simulink model "vsi_fmt_core"  (Simulink 7.0)
settings: Solver=ode45  StartTime=0.0  StopTime=10.0  RelTol=1e-3
libraries: xbsIndex_r4 x293, xbsReplacements_r4 x15, simulink x3, vlbi_lib x1
(part 1 of 2)
settings Model: Creator=mdexter  LastModifiedBy=mdexter

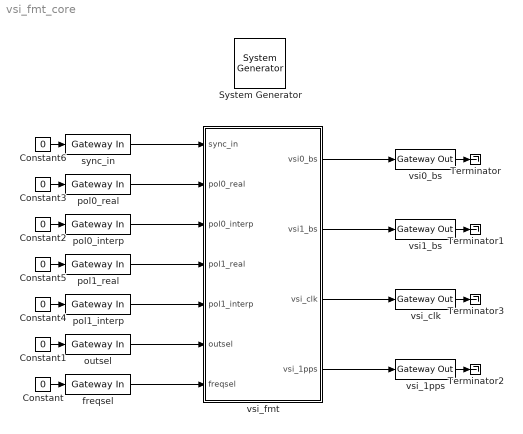
== system vsi_fmt_core ==
  " System Generator" : xbsIndex_r4/ System Generator  Tag=genX  SystemSampleTime=-1  xilinxfamily=virtex2p  part=xc2vp50  speed=-7  package=ff1152  synthesis_tool=XST  clock_wrapper=Clock Enables  directory=./vsi_fmt_core  testbench=off  simulink_period=1  sysclk_period=100  dcm_input_clock_period=100  incr_netlist=off  trim_vbits=Everywhere in SubSystem  dbl_ovrd=According to Block Masks  core_generation=According to Block Masks  run_coregen=off  deprecated_control=off  eval_field=0  block_type=sysgen
      settings: block_version=10.1.3
  Constant{,1..6} (7 alike) : Constant  Value=0
  Terminator{,1..3} (4 alike) : Terminator
  freqsel : xbsIndex_r4/Gateway In  arith_type=Unsigned  n_bits=3  bin_pt=0  quantization="Round  (unbiased: +/- Inf)"  overflow=Saturate  period=1  dbl_ovrd=off  timing_constraint=None  locs_specified=off  LOCs={}  block_type=gatewayin
      settings: infoedit="Gateway in block.  Converts inputs of type Simulink integer, double and fixed point to  Xilinx fixed point type.<P><P>Hardware notes:  In hardware these blocks become top level input ports."  block_version=10.1.3
  outsel : xbsIndex_r4/Gateway In  arith_type=Unsigned  n_bits=2  bin_pt=0  quantization="Round  (unbiased: +/- Inf)"  overflow=Saturate  period=1  dbl_ovrd=off  timing_constraint=None  locs_specified=off  LOCs={}  block_type=gatewayin
      settings: infoedit="Gateway in block.  Converts inputs of type Simulink integer, double and fixed point to  Xilinx fixed point type.<P><P>Hardware notes:  In hardware these blocks become top level input ports."  block_version=10.1.3
  pol0_interp : xbsIndex_r4/Gateway In  arith_type=Unsigned  n_bits=4  bin_pt=0  quantization="Round  (unbiased: +/- Inf)"  overflow=Saturate  period=1  dbl_ovrd=off  timing_constraint=None  locs_specified=off  LOCs={}  block_type=gatewayin
      settings: infoedit="Gateway in block.  Converts inputs of type Simulink integer, double and fixed point to  Xilinx fixed point type.<P><P>Hardware notes:  In hardware these blocks become top level input ports."  block_version=10.1.3
  pol0_real : xbsIndex_r4/Gateway In  arith_type=Unsigned  n_bits=4  bin_pt=0  quantization="Round  (unbiased: +/- Inf)"  overflow=Saturate  period=1  dbl_ovrd=off  timing_constraint=None  locs_specified=off  LOCs={}  block_type=gatewayin
      settings: infoedit="Gateway in block.  Converts inputs of type Simulink integer, double and fixed point to  Xilinx fixed point type.<P><P>Hardware notes:  In hardware these blocks become top level input ports."  block_version=10.1.3
  pol1_interp : xbsIndex_r4/Gateway In  arith_type=Unsigned  n_bits=4  bin_pt=0  quantization="Round  (unbiased: +/- Inf)"  overflow=Saturate  period=1  dbl_ovrd=off  timing_constraint=None  locs_specified=off  LOCs={}  block_type=gatewayin
      settings: infoedit="Gateway in block.  Converts inputs of type Simulink integer, double and fixed point to  Xilinx fixed point type.<P><P>Hardware notes:  In hardware these blocks become top level input ports."  block_version=10.1.3
  pol1_real : xbsIndex_r4/Gateway In  arith_type=Unsigned  n_bits=4  bin_pt=0  quantization="Round  (unbiased: +/- Inf)"  overflow=Saturate  period=1  dbl_ovrd=off  timing_constraint=None  locs_specified=off  LOCs={}  block_type=gatewayin
      settings: infoedit="Gateway in block.  Converts inputs of type Simulink integer, double and fixed point to  Xilinx fixed point type.<P><P>Hardware notes:  In hardware these blocks become top level input ports."  block_version=10.1.3
  sync_in : xbsIndex_r4/Gateway In  arith_type=Boolean  n_bits=16  bin_pt=14  quantization="Round  (unbiased: +/- Inf)"  overflow=Saturate  period=1  dbl_ovrd=off  timing_constraint=None  locs_specified=off  LOCs={}  block_type=gatewayin
      settings: infoedit="Gateway in block.  Converts inputs of type Simulink integer, double and fixed point to  Xilinx fixed point type.<P><P>Hardware notes:  In hardware these blocks become top level input ports."  block_version=10.1.3
  vsi0_bs : xbsIndex_r4/Gateway Out  hdl_port=on  timing_constraint=None  locs_specified=off  LOCs={}  block_type=gatewayout
      settings: infoedit="Gateway out block.  Converts Xilinx fixed point inputs into ouputs of type Simulink integer, double, or fixed point.<P><P>Hardware notes:  In hardware these blocks become top level output ports or are discarded, depending on how they are configured."  block_version=10.1.3
  vsi1_bs : xbsIndex_r4/Gateway Out  hdl_port=on  timing_constraint=None  locs_specified=off  LOCs={}  block_type=gatewayout
      settings: infoedit="Gateway out block.  Converts Xilinx fixed point inputs into ouputs of type Simulink integer, double, or fixed point.<P><P>Hardware notes:  In hardware these blocks become top level output ports or are discarded, depending on how they are configured."  block_version=10.1.3
  vsi_1pps : xbsIndex_r4/Gateway Out  hdl_port=on  timing_constraint=None  locs_specified=off  LOCs={}  block_type=gatewayout
      settings: infoedit="Gateway out block.  Converts Xilinx fixed point inputs into ouputs of type Simulink integer, double, or fixed point.<P><P>Hardware notes:  In hardware these blocks become top level output ports or are discarded, depending on how they are configured."  block_version=10.1.3
  vsi_clk : xbsIndex_r4/Gateway Out  hdl_port=on  timing_constraint=None  locs_specified=off  LOCs={}  block_type=gatewayout
      settings: infoedit="Gateway out block.  Converts Xilinx fixed point inputs into ouputs of type Simulink integer, double, or fixed point.<P><P>Hardware notes:  In hardware these blocks become top level output ports or are discarded, depending on how they are configured."  block_version=10.1.3
  vsi_fmt : Subsystem
  wires:
  vsi_fmt/1(vsi0_bs) -> vsi0_bs/1
  pol0_real/1 -> vsi_fmt/2(pol0_real)
  vsi_fmt/2(vsi1_bs) -> vsi1_bs/1
  pol1_real/1 -> vsi_fmt/4(pol1_real)
  pol0_interp/1 -> vsi_fmt/3(pol0_interp)
  pol1_interp/1 -> vsi_fmt/5(pol1_interp)
  sync_in/1 -> vsi_fmt/1(sync_in)
  outsel/1 -> vsi_fmt/6(outsel)
  vsi_fmt/3(vsi_clk) -> vsi_clk/1
  vsi_fmt/4(vsi_1pps) -> vsi_1pps/1
  freqsel/1 -> vsi_fmt/7(freqsel)
  Constant/1 -> freqsel/1
  Constant1/1 -> outsel/1
  Constant2/1 -> pol0_interp/1
  Constant3/1 -> pol0_real/1
  Constant4/1 -> pol1_interp/1
  Constant5/1 -> pol1_real/1
  Constant6/1 -> sync_in/1
  vsi0_bs/1 -> Terminator/1
  vsi1_bs/1 -> Terminator1/1
  vsi_1pps/1 -> Terminator2/1
  vsi_clk/1 -> Terminator3/1

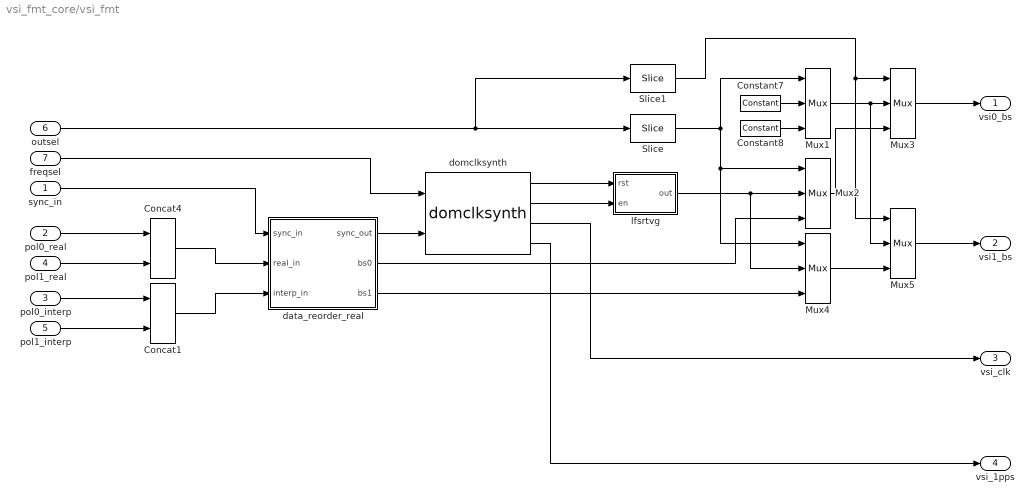
== system vsi_fmt_core/vsi_fmt ==
  sync_in : Inport  OutDataType=sfix(16)  OutScaling=2^0
  pol0_real : Inport  Port=2  OutDataType=sfix(16)  OutScaling=2^0
  pol0_interp : Inport  Port=3  OutDataType=sfix(16)  OutScaling=2^0
  pol1_real : Inport  Port=4  OutDataType=sfix(16)  OutScaling=2^0
  pol1_interp : Inport  Port=5  OutDataType=sfix(16)  OutScaling=2^0
  outsel : Inport  Port=6  OutDataType=sfix(16)  OutScaling=2^0
  freqsel : Inport  Port=7  OutDataType=sfix(16)  OutScaling=2^0
  Concat1 : xbsIndex_r4/Concat  num_inputs=2  dbl_ovrd=off  block_type=concat
      settings: block_version=11.3
  Concat4 : xbsIndex_r4/Concat  num_inputs=2  dbl_ovrd=off  block_type=concat
      settings: block_version=11.3
  Constant7 : xbsIndex_r4/Constant  arith_type=Unsigned  const=0  n_bits=32  bin_pt=0  explicit_period=on  period=1  equ=P=C  opselect=C  inp2=PCIN>>17  opr=+  inp1=P  carry=CIN  dbl_ovrd=off  block_type=constant
      settings: block_version=11.3
  Constant8 : xbsIndex_r4/Constant  arith_type=Unsigned  const=2^32-1  n_bits=32  bin_pt=0  explicit_period=on  period=1  equ=P=C  opselect=C  inp2=PCIN>>17  opr=+  inp1=P  carry=CIN  dbl_ovrd=off  block_type=constant
      settings: block_version=11.3
  Mux{1..5} (5 alike) : xbsIndex_r4/Mux  inputs=2  en=off  latency=1  precision=Full  arith_type="Signed  (2's comp)"  n_bits=8  bin_pt=2  quantization=Truncate  overflow=Wrap  dbl_ovrd=off  block_type=mux
      settings: xl_area=[0, 0, 0, 0, 0, 0, 0]  block_version=11.3
  Slice : xbsIndex_r4/Slice  nbits=1  boolean_output=off  mode=Lower Bit Location + Width  bit1=0  base1=MSB of Input  bit0=0  base0=LSB of Input  dbl_ovrd=off  block_type=slice
      settings: block_version=11.3
  Slice1 : xbsIndex_r4/Slice  nbits=1  boolean_output=off  mode=Lower Bit Location + Width  bit1=0  base1=MSB of Input  bit0=1  base0=LSB of Input  dbl_ovrd=off  block_type=slice
      settings: block_version=11.3
  data_reorder_real : Subsystem  mask{sample_width=2, vsi_clock=64 MHz}
      mask prompts: sample_width "Channel sample width:"; vsi_clock "VSI output clock rate:"
      mask init:
      | myname = gcb;
      | 
      | if (strcmp(vsi_clock, '32 MHz'))
      |     set_param([gcb, '/restream'], 'clock_rate', '32');
      |     set_param([gcb, '/slc_wrmask'], 'bit1', '-1');
      | else
      |     set_param([gcb, '/restream'], 'clock_rate', '64');
      |     set_param([gcb, '/slc_wrmask'], 'bit1', '0');
      | end
      mask StyleString: edit,popup(32 MHz|64 MHz)
  domclksynth : vlbi_lib/domclksynth  SystemSampleTime=-1
  lfsrtvg : Subsystem
  vsi0_bs : Outport  OutDataType=sfix(16)  OutScaling=2^0
  vsi1_bs : Outport  Port=2  OutDataType=sfix(16)  OutScaling=2^0
  vsi_clk : Outport  Port=3  OutDataType=sfix(16)  OutScaling=2^0
  vsi_1pps : Outport  Port=4  OutDataType=sfix(16)  OutScaling=2^0
  wires:
  domclksynth/2 -> lfsrtvg/2(en)
  domclksynth/3 -> vsi_clk/1
  domclksynth/4 -> vsi_1pps/1
  data_reorder_real/1(sync_out) -> domclksynth/2
  data_reorder_real/2(bs0) -> Mux2/3
  domclksynth/1 -> lfsrtvg/1(rst)
  outsel/1 -> Slice/1, Slice1/1
  Constant7/1 -> Mux1/2
  Constant8/1 -> Mux1/3
  Slice/1 -> Mux1/1, Mux2/1, Mux4/1
  lfsrtvg/1(out) -> Mux2/2, Mux4/2
  Mux1/1 -> Mux3/2, Mux5/2
  Mux2/1 -> Mux3/3
  Slice1/1 -> Mux3/1, Mux5/1
  Concat4/1 -> data_reorder_real/2(real_in)
  Concat1/1 -> data_reorder_real/3(interp_in)
  data_reorder_real/3(bs1) -> Mux4/3
  Mux4/1 -> Mux5/3
  pol0_real/1 -> Concat4/1
  pol1_real/1 -> Concat4/2
  pol0_interp/1 -> Concat1/1
  pol1_interp/1 -> Concat1/2
  sync_in/1 -> data_reorder_real/1(sync_in)
  Mux3/1 -> vsi0_bs/1
  Mux5/1 -> vsi1_bs/1
  freqsel/1 -> domclksynth/1

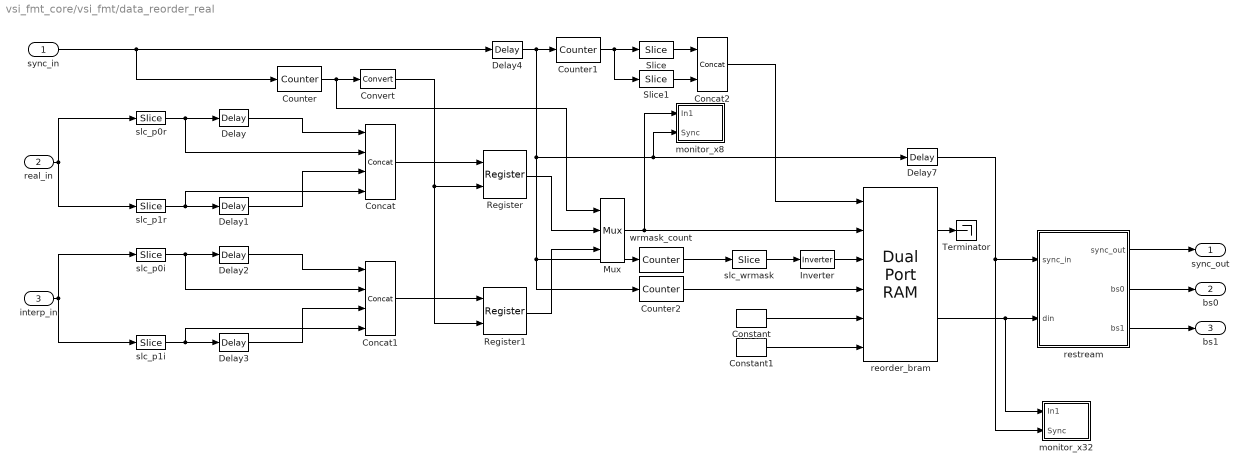
== system vsi_fmt_core/vsi_fmt/data_reorder_real ==
  sync_in : Inport  OutDataType=sfix(16)  OutScaling=2^0
  real_in : Inport  Port=2  OutDataType=sfix(16)  OutScaling=2^0
  interp_in : Inport  Port=3  OutDataType=sfix(16)  OutScaling=2^0
  Concat : xbsIndex_r4/Concat  num_inputs=4  dbl_ovrd=off  block_type=concat
      settings: block_version=11.3
  Concat1 : xbsIndex_r4/Concat  num_inputs=4  dbl_ovrd=off  block_type=concat
      settings: block_version=11.3
  Concat2 : xbsIndex_r4/Concat  num_inputs=2  dbl_ovrd=off  block_type=concat
      settings: block_version=11.3
  Constant : xbsIndex_r4/Constant  arith_type=Unsigned  const=0  n_bits=32*sample_width  bin_pt=0  explicit_period=on  period=1  equ=P=C  opselect=C  inp2=PCIN>>17  opr=+  inp1=P  carry=CIN  dbl_ovrd=off  block_type=constant
      settings: block_version=11.3
  Constant1 : xbsIndex_r4/Constant  arith_type=Boolean  const=0  n_bits=8*sample_width  bin_pt=0  explicit_period=on  period=1  equ=P=C  opselect=C  inp2=PCIN>>17  opr=+  inp1=P  carry=CIN  dbl_ovrd=off  block_type=constant
      settings: block_version=11.3
  Convert : xbsIndex_r4/Convert  arith_type=Boolean  n_bits=8  bin_pt=6  quantization=Truncate  overflow=Wrap  latency=0  dbl_ovrd=off  pipeline=off  block_type=convert
      settings: xl_area=[0, 0, 0, 0, 0, 0, 0]  block_version=11.3
  Counter : xbsIndex_r4/Counter  cnt_type=Free Running  cnt_to=Inf  operation=Up  start_count=0  cnt_by_val=1  arith_type=Unsigned  n_bits=1  bin_pt=0  load_pin=off  rst=on  en=off  explicit_period=off  period=1  dbl_ovrd=off  use_behavioral_HDL=off  use_rpm=on  implementation=Fabric  block_type=counter
      settings: xl_area=[0, 0, 0, 0, 0, 0, 0]  block_version=11.3
  Counter1 : xbsIndex_r4/Counter  cnt_type=Free Running  cnt_to=Inf  operation=Up  start_count=0  cnt_by_val=1  arith_type=Unsigned  n_bits=3  bin_pt=0  load_pin=off  rst=on  en=off  explicit_period=off  period=1  dbl_ovrd=off  use_behavioral_HDL=off  use_rpm=on  implementation=Fabric  block_type=counter
      settings: xl_area=[0, 0, 0, 0, 0, 0, 0]  block_version=11.3
  Counter2 : xbsIndex_r4/Counter  cnt_type=Free Running  cnt_to=Inf  operation=Up  start_count=0  cnt_by_val=1  arith_type=Unsigned  n_bits=1  bin_pt=0  load_pin=off  rst=on  en=off  explicit_period=off  period=1  dbl_ovrd=off  use_behavioral_HDL=off  use_rpm=on  implementation=Fabric  block_type=counter
      settings: xl_area=[0, 0, 0, 0, 0, 0, 0]  block_version=11.3
  Delay{,1..3} (4 alike) : xbsIndex_r4/Delay  en=off  latency=1  dbl_ovrd=off  reg_retiming=off  block_type=delay
      settings: xl_area=[0, 0, 0, 0, 0, 0, 0]  block_version=11.3
  Delay4 : xbsIndex_r4/Delay  en=off  latency=3  dbl_ovrd=off  reg_retiming=off  block_type=delay
      settings: xl_area=[0, 0, 0, 0, 0, 0, 0]  block_version=11.3
  Delay7 : xbsIndex_r4/Delay  en=off  latency=11  dbl_ovrd=off  reg_retiming=off  block_type=delay
      settings: xl_area=[0, 0, 0, 0, 0, 0, 0]  block_version=11.3
  Inverter : xbsIndex_r4/Inverter  en=off  latency=0  dbl_ovrd=off  block_type=inv
      settings: xl_area=[0, 0, 0, 0, 0, 0, 0]  block_version=11.3
  Mux : xbsIndex_r4/Mux  inputs=2  en=off  latency=1  precision=Full  arith_type="Signed  (2's comp)"  n_bits=8  bin_pt=2  quantization=Truncate  overflow=Wrap  dbl_ovrd=off  block_type=mux
      settings: xl_area=[0, 0, 0, 0, 0, 0, 0]  block_version=11.3
  Register : xbsIndex_r4/Register  init=0  rst=off  en=on  dbl_ovrd=off  block_type=register
      settings: xl_area=[0, 0, 0, 0, 0, 0, 0]  block_version=11.3
  Register1 : xbsIndex_r4/Register  init=0  rst=off  en=on  dbl_ovrd=off  block_type=register
      settings: xl_area=[0, 0, 0, 0, 0, 0, 0]  block_version=11.3
  Slice : xbsIndex_r4/Slice  nbits=1  boolean_output=off  mode=Lower Bit Location + Width  bit1=0  base1=MSB of Input  bit0=0  base0=LSB of Input  dbl_ovrd=off  block_type=slice
      settings: block_version=11.3
  Slice1 : xbsIndex_r4/Slice  nbits=2  boolean_output=off  mode=Upper Bit Location + Width  bit1=0  base1=MSB of Input  bit0=0  base0=LSB of Input  dbl_ovrd=off  block_type=slice
      settings: block_version=11.3
  Terminator : Terminator
  monitor_x32 : Subsystem
  monitor_x8 : Subsystem
  reorder_bram : xbsIndex_r4/Dual Port RAM  depth=8  initVector=zeros(2)  distributed_mem=Block RAM  init_a=0  init_b=0  rst_a=off  rst_b=off  en_a=off  en_b=off  latency=3  write_mode_A=Read Before Write  write_mode_B=Read Before Write  dbl_ovrd=off  optimize=Area  use_rpm=off  block_type=dpram
      settings: xl_area=[0, 0, 0, 0, 0, 0, 0]  block_version=11.3
  restream : Subsystem  mask{clock_rate=64}
      mask prompts: clock_rate "Clock rate (MHz)"
  slc_p0i : xbsIndex_r4/Slice  nbits=2*sample_width  boolean_output=off  mode=Upper Bit Location + Width  bit1=0  base1=MSB of Input  bit0=0  base0=LSB of Input  dbl_ovrd=off  block_type=slice
      settings: block_version=11.3
  slc_p0r : xbsIndex_r4/Slice  nbits=2*sample_width  boolean_output=off  mode=Upper Bit Location + Width  bit1=0  base1=MSB of Input  bit0=0  base0=LSB of Input  dbl_ovrd=off  block_type=slice
      settings: block_version=11.3
  slc_p1i : xbsIndex_r4/Slice  nbits=2*sample_width  boolean_output=off  mode=Upper Bit Location + Width  bit1=-2*sample_width  base1=MSB of Input  bit0=0  base0=LSB of Input  dbl_ovrd=off  block_type=slice
      settings: block_version=11.3
  slc_p1r : xbsIndex_r4/Slice  nbits=2*sample_width  boolean_output=off  mode=Upper Bit Location + Width  bit1=-2*sample_width  base1=MSB of Input  bit0=0  base0=LSB of Input  dbl_ovrd=off  block_type=slice
      settings: block_version=11.3
  slc_wrmask : xbsIndex_r4/Slice  nbits=1  boolean_output=on  mode=Upper Bit Location + Width  bit1=0  base1=MSB of Input  bit0=0  base0=LSB of Input  dbl_ovrd=off  block_type=slice
      settings: block_version=11.3
  wrmask_count : xbsIndex_r4/Counter  cnt_type=Count Limited  cnt_to=31  operation=Up  start_count=0  cnt_by_val=1  arith_type=Unsigned  n_bits=6  bin_pt=0  load_pin=off  rst=on  en=off  explicit_period=off  period=1  dbl_ovrd=off  use_behavioral_HDL=off  use_rpm=on  implementation=Fabric  block_type=counter
      settings: xl_area=[0, 0, 0, 0, 0, 0, 0]  block_version=11.3
  sync_out : Outport  OutDataType=sfix(16)  OutScaling=2^0
  bs0 : Outport  Port=2  OutDataType=sfix(16)  OutScaling=2^0
  bs1 : Outport  Port=3  OutDataType=sfix(16)  OutScaling=2^0
  wires:
  Inverter/1 -> reorder_bram/3
  wrmask_count/1 -> slc_wrmask/1
  restream/3(bs1) -> bs1/1
  restream/2(bs0) -> bs0/1
  restream/1(sync_out) -> sync_out/1
  reorder_bram/2 -> monitor_x32/1(In1), restream/2(din)
  Delay7/1 -> monitor_x32/2(Sync), restream/1(sync_in)
  Concat2/1 -> reorder_bram/1
  Counter1/1 -> Slice1/1, Slice/1
  Slice1/1 -> Concat2/2
  Slice/1 -> Concat2/1
  reorder_bram/1 -> Terminator/1
  Counter2/1 -> reorder_bram/4
  Delay4/1 -> wrmask_count/1, Counter2/1, monitor_x8/2(Sync), Delay7/1, Counter1/1
  slc_wrmask/1 -> Inverter/1
  Mux/1 -> reorder_bram/2, monitor_x8/1(In1)
  Constant1/1 -> reorder_bram/6
  Constant/1 -> reorder_bram/5
  Register1/1 -> Mux/3
  Register/1 -> Mux/2
  Convert/1 -> Register1/2, Register/2
  Counter/1 -> Mux/1, Convert/1
  sync_in/1 -> Delay4/1, Counter/1
  Concat1/1 -> Register1/1
  Concat/1 -> Register/1
  Delay3/1 -> Concat1/3
  Delay2/1 -> Concat1/1
  Delay1/1 -> Concat/3
  Delay/1 -> Concat/1
  slc_p1i/1 -> Concat1/4, Delay3/1
  slc_p0i/1 -> Concat1/2, Delay2/1
  slc_p1r/1 -> Concat/4, Delay1/1
  slc_p0r/1 -> Concat/2, Delay/1
  interp_in/1 -> slc_p1i/1, slc_p0i/1
  real_in/1 -> slc_p1r/1, slc_p0r/1

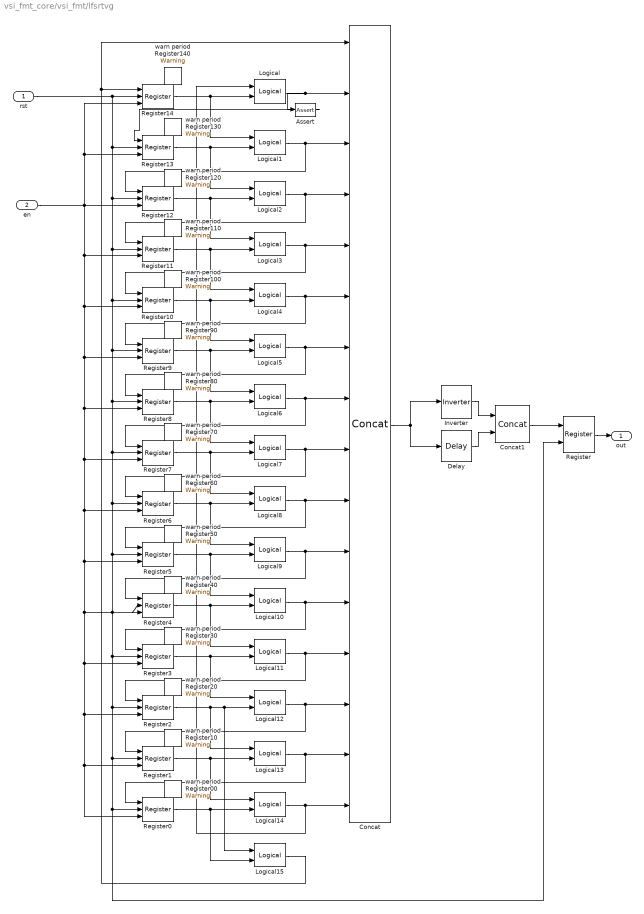
== system vsi_fmt_core/vsi_fmt/lfsrtvg ==
  rst : Inport  OutDataType=sfix(16)  OutScaling=2^0
  en : Inport  Port=2  OutDataType=sfix(16)  OutScaling=2^0
  Assert : xbsIndex_r4/Assert  assert_type=on  type_source=Explicitly  arith_type=Boolean  n_bits=16  bin_pt=14  assert_rate=on  rate_source=Explicitly  period=1  output_port=on  block_type=assert
      settings: block_version=11.3
  Concat : xbsIndex_r4/Concat  num_inputs=16  dbl_ovrd=off  block_type=concat
      settings: block_version=11.3
  Concat1 : xbsIndex_r4/Concat  num_inputs=2  dbl_ovrd=off  block_type=concat
      settings: block_version=11.3
  Delay : xbsIndex_r4/Delay  en=off  latency=0  dbl_ovrd=off  reg_retiming=off  block_type=delay
      settings: xl_area=[0, 0, 0, 0, 0, 0, 0]  block_version=11.3
  Inverter : xbsIndex_r4/Inverter  en=off  latency=0  dbl_ovrd=off  block_type=inv
      settings: xl_area=[0, 0, 0, 0, 0, 0, 0]  block_version=11.3
  Logical{,1..15} (16 alike) : xbsIndex_r4/Logical  logical_function=XOR  inputs=2  en=off  latency=0  precision=Full  arith_type=Unsigned  n_bits=8  bin_pt=2  align_bp=on  dbl_ovrd=off  block_type=logical
      settings: xl_area=[0, 0, 0, 0, 0, 0, 0]  block_version=11.3
  Register : xbsIndex_r4/Register  init=3221176320  rst=on  en=off  dbl_ovrd=off  block_type=register
      settings: xl_area=[0, 0, 0, 0, 0, 0, 0]  block_version=11.3
  Register{0..14} (15 alike) : xbsIndex_r4/Register  init=1  rst=on  en=on  dbl_ovrd=off  block_type=register
      settings: xl_area=[0, 0, 0, 0, 0, 0, 0]  block_version=11.3
  warn period Register00 : xbsReplacements_r4/Warning  SystemSampleTime=-1  period=1
  warn period Register{10,20,30,40,50,60,70,80,90,100,110,120,130,140} (14 alike) : xbsReplacements_r4/Warning  SystemSampleTime=-1  period=1
  out : Outport  OutDataType=sfix(16)  OutScaling=2^0
  wires:
  en/1 -> Register9/3, Register8/3, Register0/3, Register1/3, Register2/3, Register3/3, Register4/3, Register5/3, Register6/3, Register7/3, Register10/3, Register11/3, Register12/3, Register13/3, Register14/3
  rst/1 -> Register13/2, Register12/2, Register11/2, Register10/2, Register9/2, Register8/2, Register7/2, Register6/2, Register5/2, Register4/2, Register3/2, Register2/2, Register1/2, Register0/2, Register/2, Register14/2
  Register14/1 -> Logical1/1, Logical/2
  Register13/1 -> Logical2/1, Logical1/2
  Register12/1 -> Logical3/1, Logical2/2
  Register11/1 -> Logical4/1, Logical3/2
  Register10/1 -> Logical5/1, Logical4/2
  Register9/1 -> Logical6/1, Logical5/2
  Register8/1 -> Logical7/1, Logical6/2
  Register7/1 -> Logical8/1, Logical7/2
  Register6/1 -> Logical9/1, Logical8/2
  Register5/1 -> Logical10/1, Logical9/2
  Register4/1 -> Logical11/1, Logical10/2
  Register3/1 -> Logical12/1, Logical11/2
  Register2/1 -> Logical13/1, Logical12/2, Logical15/1
  Register1/1 -> Logical14/1, Logical13/2
  Register0/1 -> Logical14/2, Logical15/2
  Logical14/1 -> Logical/1, Concat/16
  Logical15/1 -> Register14/1, Concat/1
  Logical/1 -> Concat/2, Assert/1
  Logical1/1 -> Register12/1, Concat/3
  Logical2/1 -> Register11/1, Concat/4
  Logical3/1 -> Register10/1, Concat/5
  Logical4/1 -> Register9/1, Concat/6
  Logical5/1 -> Register8/1, Concat/7
  Logical6/1 -> Register7/1, Concat/8
  Logical7/1 -> Register6/1, Concat/9
  Logical8/1 -> Register5/1, Concat/10
  Logical9/1 -> Register4/1, Concat/11
  Logical10/1 -> Register3/1, Concat/12
  Logical11/1 -> Register2/1, Concat/13
  Logical12/1 -> Register1/1, Concat/14
  Logical13/1 -> Register0/1, Concat/15
  Concat/1 -> Inverter/1, Delay/1
  Inverter/1 -> Concat1/1
  Delay/1 -> Concat1/2
  Concat1/1 -> Register/1
  Register/1 -> out/1
  Assert/1 -> Register13/1

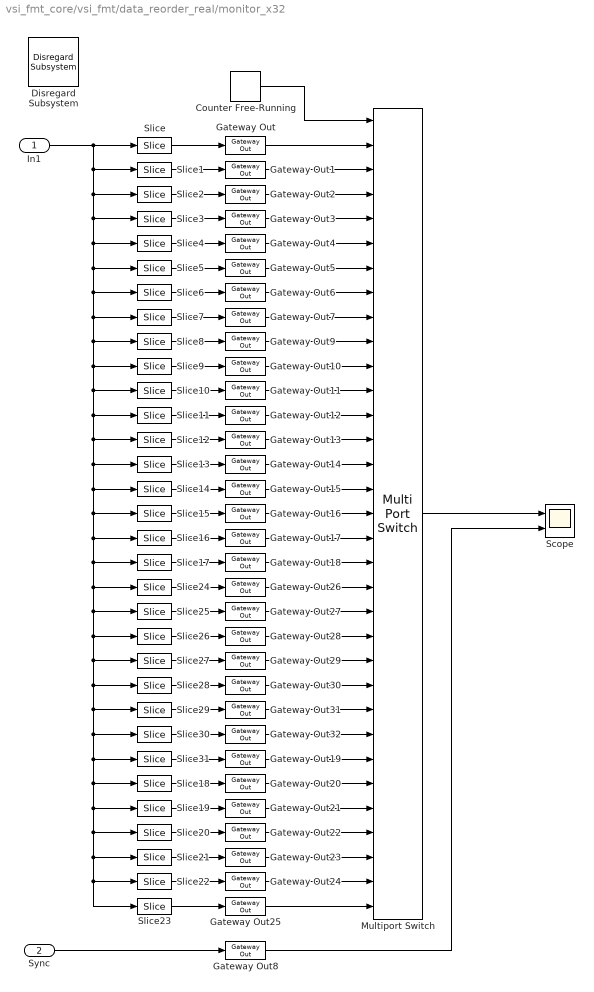
== system vsi_fmt_core/vsi_fmt/data_reorder_real/monitor_x32 ==
  In1 : Inport  OutDataType=sfix(16)  OutScaling=2^0
  Sync : Inport  Port=2  OutDataType=sfix(16)  OutScaling=2^0
  Counter Free-Running : simulink/Sources/Counter Free-Running  SystemSampleTime=-1  NumBits=5  tsamp=1/32
  Disregard Subsystem : xbsIndex_r4/Disregard Subsystem  Tag=discardX  block_type=disregard
      settings: block_version=11.3
  Gateway Out{,1..32} (33 alike) : xbsIndex_r4/Gateway Out  hdl_port=off  timing_constraint=None  locs_specified=off  LOCs={}  block_type=gatewayout
      settings: infoedit="Gateway out block.  Converts Xilinx fixed point inputs into ouputs of type Simulink integer, double, or fixed point.<br><br>Hardware notes:  In hardware these blocks become top level output ports or are discarded, depending on how they are configured."  xl_area=[0, 0, 0, 0, 0, 0, 0]  block_version=11.3
  Multiport Switch : MultiPortSwitch  Inputs=32  zeroidx=on  SampleTime=1/32
  Scope : Scope  NumInputPorts=2
      settings: YMin=-5~-5  YMax=5~5
  Slice : xbsIndex_r4/Slice  nbits=sample_width  boolean_output=off  mode=Lower Bit Location + Width  bit1=sample_width*0  base1=MSB of Input  bit0=sample_width*7  base0=LSB of Input  dbl_ovrd=off  block_type=slice
      settings: block_version=11.3
  Slice1 : xbsIndex_r4/Slice  nbits=sample_width  boolean_output=off  mode=Lower Bit Location + Width  bit1=-2*sample_width  base1=MSB of Input  bit0=sample_width*6  base0=LSB of Input  dbl_ovrd=off  block_type=slice
      settings: block_version=11.3
  Slice10 : xbsIndex_r4/Slice  nbits=sample_width  boolean_output=off  mode=Lower Bit Location + Width  bit1=sample_width*21  base1=MSB of Input  bit0=sample_width*21  base0=LSB of Input  dbl_ovrd=off  block_type=slice
      settings: block_version=11.3
  Slice11 : xbsIndex_r4/Slice  nbits=sample_width  boolean_output=off  mode=Lower Bit Location + Width  bit1=-22*sample_width  base1=MSB of Input  bit0=sample_width*20  base0=LSB of Input  dbl_ovrd=off  block_type=slice
      settings: block_version=11.3
  Slice12 : xbsIndex_r4/Slice  nbits=sample_width  boolean_output=off  mode=Lower Bit Location + Width  bit1=-24*sample_width  base1=MSB of Input  bit0=sample_width*31  base0=LSB of Input  dbl_ovrd=off  block_type=slice
      settings: block_version=11.3
  Slice13 : xbsIndex_r4/Slice  nbits=sample_width  boolean_output=off  mode=Lower Bit Location + Width  bit1=-26*sample_width  base1=MSB of Input  bit0=sample_width*30  base0=LSB of Input  dbl_ovrd=off  block_type=slice
      settings: block_version=11.3
  Slice14 : xbsIndex_r4/Slice  nbits=sample_width  boolean_output=off  mode=Lower Bit Location + Width  bit1=-28*sample_width  base1=MSB of Input  bit0=sample_width*29  base0=LSB of Input  dbl_ovrd=off  block_type=slice
      settings: block_version=11.3
  Slice15 : xbsIndex_r4/Slice  nbits=sample_width  boolean_output=off  mode=Lower Bit Location + Width  bit1=-30*sample_width  base1=MSB of Input  bit0=sample_width*28  base0=LSB of Input  dbl_ovrd=off  block_type=slice
      settings: block_version=11.3
  Slice16 : xbsIndex_r4/Slice  nbits=sample_width  boolean_output=off  mode=Lower Bit Location + Width  bit1=-1*sample_width  base1=MSB of Input  bit0=sample_width*3  base0=LSB of Input  dbl_ovrd=off  block_type=slice
      settings: block_version=11.3
  Slice17 : xbsIndex_r4/Slice  nbits=sample_width  boolean_output=off  mode=Lower Bit Location + Width  bit1=-3*sample_width  base1=MSB of Input  bit0=sample_width*2  base0=LSB of Input  dbl_ovrd=off  block_type=slice
      settings: block_version=11.3
  Slice18 : xbsIndex_r4/Slice  nbits=sample_width  boolean_output=off  mode=Lower Bit Location + Width  bit1=-21*sample_width  base1=MSB of Input  bit0=sample_width*17  base0=LSB of Input  dbl_ovrd=off  block_type=slice
      settings: block_version=11.3
  Slice19 : xbsIndex_r4/Slice  nbits=sample_width  boolean_output=off  mode=Lower Bit Location + Width  bit1=-23*sample_width  base1=MSB of Input  bit0=sample_width*16  base0=LSB of Input  dbl_ovrd=off  block_type=slice
      settings: block_version=11.3
  Slice2 : xbsIndex_r4/Slice  nbits=sample_width  boolean_output=off  mode=Lower Bit Location + Width  bit1=-4*sample_width  base1=MSB of Input  bit0=sample_width*5  base0=LSB of Input  dbl_ovrd=off  block_type=slice
      settings: block_version=11.3
  Slice20 : xbsIndex_r4/Slice  nbits=sample_width  boolean_output=off  mode=Lower Bit Location + Width  bit1=-25*sample_width  base1=MSB of Input  bit0=sample_width*27  base0=LSB of Input  dbl_ovrd=off  block_type=slice
      settings: block_version=11.3
  Slice21 : xbsIndex_r4/Slice  nbits=sample_width  boolean_output=off  mode=Lower Bit Location + Width  bit1=-27*sample_width  base1=MSB of Input  bit0=sample_width*26  base0=LSB of Input  dbl_ovrd=off  block_type=slice
      settings: block_version=11.3
  Slice22 : xbsIndex_r4/Slice  nbits=sample_width  boolean_output=off  mode=Lower Bit Location + Width  bit1=-29*sample_width  base1=MSB of Input  bit0=sample_width*25  base0=LSB of Input  dbl_ovrd=off  block_type=slice
      settings: block_version=11.3
  Slice23 : xbsIndex_r4/Slice  nbits=sample_width  boolean_output=off  mode=Lower Bit Location + Width  bit1=-31*sample_width  base1=MSB of Input  bit0=sample_width*24  base0=LSB of Input  dbl_ovrd=off  block_type=slice
      settings: block_version=11.3
  Slice24 : xbsIndex_r4/Slice  nbits=sample_width  boolean_output=off  mode=Lower Bit Location + Width  bit1=-5*sample_width  base1=MSB of Input  bit0=sample_width*1  base0=LSB of Input  dbl_ovrd=off  block_type=slice
      settings: block_version=11.3
  Slice25 : xbsIndex_r4/Slice  nbits=sample_width  boolean_output=off  mode=Lower Bit Location + Width  bit1=-7*sample_width  base1=MSB of Input  bit0=sample_width*0  base0=LSB of Input  dbl_ovrd=off  block_type=slice
      settings: block_version=11.3
  Slice26 : xbsIndex_r4/Slice  nbits=sample_width  boolean_output=off  mode=Lower Bit Location + Width  bit1=-9*sample_width  base1=MSB of Input  bit0=sample_width*11  base0=LSB of Input  dbl_ovrd=off  block_type=slice
      settings: block_version=11.3
  Slice27 : xbsIndex_r4/Slice  nbits=sample_width  boolean_output=off  mode=Lower Bit Location + Width  bit1=-11*sample_width  base1=MSB of Input  bit0=sample_width*10  base0=LSB of Input  dbl_ovrd=off  block_type=slice
      settings: block_version=11.3
  Slice28 : xbsIndex_r4/Slice  nbits=sample_width  boolean_output=off  mode=Lower Bit Location + Width  bit1=-13*sample_width  base1=MSB of Input  bit0=sample_width*9  base0=LSB of Input  dbl_ovrd=off  block_type=slice
      settings: block_version=11.3
  Slice29 : xbsIndex_r4/Slice  nbits=sample_width  boolean_output=off  mode=Lower Bit Location + Width  bit1=-15*sample_width  base1=MSB of Input  bit0=sample_width*8  base0=LSB of Input  dbl_ovrd=off  block_type=slice
      settings: block_version=11.3
  Slice3 : xbsIndex_r4/Slice  nbits=sample_width  boolean_output=off  mode=Lower Bit Location + Width  bit1=-6*sample_width  base1=MSB of Input  bit0=sample_width*4  base0=LSB of Input  dbl_ovrd=off  block_type=slice
      settings: block_version=11.3
  Slice30 : xbsIndex_r4/Slice  nbits=sample_width  boolean_output=off  mode=Lower Bit Location + Width  bit1=-17*sample_width  base1=MSB of Input  bit0=sample_width*19  base0=LSB of Input  dbl_ovrd=off  block_type=slice
      settings: block_version=11.3
  Slice31 : xbsIndex_r4/Slice  nbits=sample_width  boolean_output=off  mode=Lower Bit Location + Width  bit1=sample_width*18  base1=MSB of Input  bit0=sample_width*18  base0=LSB of Input  dbl_ovrd=off  block_type=slice
      settings: block_version=11.3
  Slice4 : xbsIndex_r4/Slice  nbits=sample_width  boolean_output=off  mode=Lower Bit Location + Width  bit1=-8*sample_width  base1=MSB of Input  bit0=sample_width*15  base0=LSB of Input  dbl_ovrd=off  block_type=slice
      settings: block_version=11.3
  Slice5 : xbsIndex_r4/Slice  nbits=sample_width  boolean_output=off  mode=Lower Bit Location + Width  bit1=-10*sample_width  base1=MSB of Input  bit0=sample_width*14  base0=LSB of Input  dbl_ovrd=off  block_type=slice
      settings: block_version=11.3
  Slice6 : xbsIndex_r4/Slice  nbits=sample_width  boolean_output=off  mode=Lower Bit Location + Width  bit1=-12*sample_width  base1=MSB of Input  bit0=sample_width*13  base0=LSB of Input  dbl_ovrd=off  block_type=slice
      settings: block_version=11.3
  Slice7 : xbsIndex_r4/Slice  nbits=sample_width  boolean_output=off  mode=Lower Bit Location + Width  bit1=-14*sample_width  base1=MSB of Input  bit0=sample_width*12  base0=LSB of Input  dbl_ovrd=off  block_type=slice
      settings: block_version=11.3
  Slice8 : xbsIndex_r4/Slice  nbits=sample_width  boolean_output=off  mode=Lower Bit Location + Width  bit1=-16*sample_width  base1=MSB of Input  bit0=sample_width*23  base0=LSB of Input  dbl_ovrd=off  block_type=slice
      settings: block_version=11.3
  Slice9 : xbsIndex_r4/Slice  nbits=sample_width  boolean_output=off  mode=Lower Bit Location + Width  bit1=-18*sample_width  base1=MSB of Input  bit0=sample_width*22  base0=LSB of Input  dbl_ovrd=off  block_type=slice
      settings: block_version=11.3
  wires:
  Gateway Out25/1 -> Multiport Switch/33
  Gateway Out24/1 -> Multiport Switch/32
  Gateway Out23/1 -> Multiport Switch/31
  Gateway Out22/1 -> Multiport Switch/30
  Gateway Out21/1 -> Multiport Switch/29
  Gateway Out20/1 -> Multiport Switch/28
  Gateway Out19/1 -> Multiport Switch/27
  Gateway Out32/1 -> Multiport Switch/26
  Gateway Out31/1 -> Multiport Switch/25
  Gateway Out30/1 -> Multiport Switch/24
  Gateway Out29/1 -> Multiport Switch/23
  Gateway Out28/1 -> Multiport Switch/22
  Gateway Out27/1 -> Multiport Switch/21
  Gateway Out26/1 -> Multiport Switch/20
  Gateway Out18/1 -> Multiport Switch/19
  Gateway Out17/1 -> Multiport Switch/18
  Gateway Out16/1 -> Multiport Switch/17
  Gateway Out15/1 -> Multiport Switch/16
  Gateway Out14/1 -> Multiport Switch/15
  Gateway Out13/1 -> Multiport Switch/14
  Gateway Out12/1 -> Multiport Switch/13
  Gateway Out11/1 -> Multiport Switch/12
  Gateway Out10/1 -> Multiport Switch/11
  Gateway Out9/1 -> Multiport Switch/10
  Gateway Out7/1 -> Multiport Switch/9
  Gateway Out6/1 -> Multiport Switch/8
  Gateway Out5/1 -> Multiport Switch/7
  Gateway Out4/1 -> Multiport Switch/6
  Gateway Out3/1 -> Multiport Switch/5
  Gateway Out2/1 -> Multiport Switch/4
  Gateway Out1/1 -> Multiport Switch/3
  Gateway Out/1 -> Multiport Switch/2
  Slice30/1 -> Gateway Out32/1
  Slice31/1 -> Gateway Out19/1
  Slice18/1 -> Gateway Out20/1
  Slice19/1 -> Gateway Out21/1
  Slice20/1 -> Gateway Out22/1
  Slice21/1 -> Gateway Out23/1
  Slice22/1 -> Gateway Out24/1
  Slice23/1 -> Gateway Out25/1
  Slice16/1 -> Gateway Out17/1
  Slice17/1 -> Gateway Out18/1
  Slice24/1 -> Gateway Out26/1
  Slice25/1 -> Gateway Out27/1
  Slice26/1 -> Gateway Out28/1
  Slice27/1 -> Gateway Out29/1
  Slice28/1 -> Gateway Out30/1
  Slice29/1 -> Gateway Out31/1
  Slice8/1 -> Gateway Out9/1
  Slice9/1 -> Gateway Out10/1
  Slice10/1 -> Gateway Out11/1
  Slice11/1 -> Gateway Out12/1
  Slice12/1 -> Gateway Out13/1
  Slice13/1 -> Gateway Out14/1
  Slice14/1 -> Gateway Out15/1
  Slice15/1 -> Gateway Out16/1
  In1/1 -> Slice/1, Slice1/1, Slice2/1, Slice3/1, Slice4/1, Slice5/1, Slice8/1, Slice9/1, Slice10/1, Slice11/1, Slice12/1, Slice13/1, Slice28/1, Slice29/1, Slice23/1, Slice22/1, Slice21/1, Slice20/1, Slice19/1, Slice18/1, Slice31/1, Slice30/1, Slice27/1, Slice26/1, Slice25/1, Slice24/1, Slice17/1, Slice16/1, Slice15/1, Slice14/1, Slice7/1, Slice6/1
  Slice/1 -> Gateway Out/1
  Slice1/1 -> Gateway Out1/1
  Slice2/1 -> Gateway Out2/1
  Slice3/1 -> Gateway Out3/1
  Slice4/1 -> Gateway Out4/1
  Slice5/1 -> Gateway Out5/1
  Slice6/1 -> Gateway Out6/1
  Slice7/1 -> Gateway Out7/1
  Counter Free-Running/1 -> Multiport Switch/1
  Multiport Switch/1 -> Scope/1
  Sync/1 -> Gateway Out8/1
  Gateway Out8/1 -> Scope/2

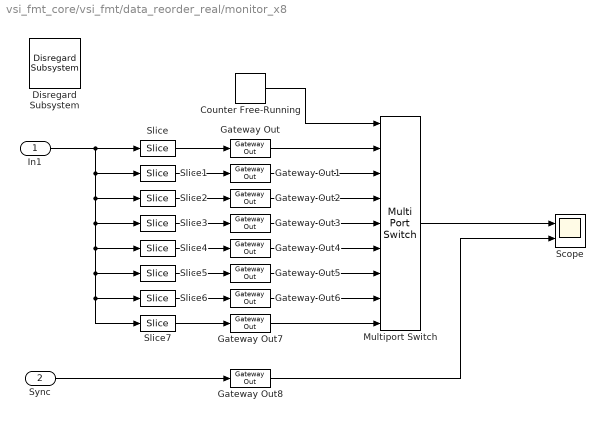
== system vsi_fmt_core/vsi_fmt/data_reorder_real/monitor_x8 ==
  In1 : Inport  OutDataType=sfix(16)  OutScaling=2^0
  Sync : Inport  Port=2  OutDataType=sfix(16)  OutScaling=2^0
  Counter Free-Running : simulink/Sources/Counter Free-Running  SystemSampleTime=-1  NumBits=3  tsamp=1/8
  Disregard Subsystem : xbsIndex_r4/Disregard Subsystem  Tag=discardX  block_type=disregard
      settings: block_version=11.3
  Gateway Out{,1..8} (9 alike) : xbsIndex_r4/Gateway Out  hdl_port=off  timing_constraint=None  locs_specified=off  LOCs={}  block_type=gatewayout
      settings: infoedit="Gateway out block.  Converts Xilinx fixed point inputs into ouputs of type Simulink integer, double, or fixed point.<br><br>Hardware notes:  In hardware these blocks become top level output ports or are discarded, depending on how they are configured."  xl_area=[0, 0, 0, 0, 0, 0, 0]  block_version=11.3
  Multiport Switch : MultiPortSwitch  Inputs=8  zeroidx=on  SampleTime=1/8
  Scope : Scope  NumInputPorts=2
      settings: YMin=-5~-5  YMax=5~5
  Slice : xbsIndex_r4/Slice  nbits=sample_width  boolean_output=off  mode=Upper Bit Location + Width  bit1=0  base1=MSB of Input  bit0=0  base0=LSB of Input  dbl_ovrd=off  block_type=slice
      settings: block_version=11.3
  Slice1 : xbsIndex_r4/Slice  nbits=sample_width  boolean_output=off  mode=Upper Bit Location + Width  bit1=-1*sample_width  base1=MSB of Input  bit0=0  base0=LSB of Input  dbl_ovrd=off  block_type=slice
      settings: block_version=11.3
  Slice2 : xbsIndex_r4/Slice  nbits=sample_width  boolean_output=off  mode=Upper Bit Location + Width  bit1=-2*sample_width  base1=MSB of Input  bit0=0  base0=LSB of Input  dbl_ovrd=off  block_type=slice
      settings: block_version=11.3
  Slice3 : xbsIndex_r4/Slice  nbits=sample_width  boolean_output=off  mode=Upper Bit Location + Width  bit1=-3*sample_width  base1=MSB of Input  bit0=0  base0=LSB of Input  dbl_ovrd=off  block_type=slice
      settings: block_version=11.3
  Slice4 : xbsIndex_r4/Slice  nbits=sample_width  boolean_output=off  mode=Upper Bit Location + Width  bit1=-4*sample_width  base1=MSB of Input  bit0=0  base0=LSB of Input  dbl_ovrd=off  block_type=slice
      settings: block_version=11.3
  Slice5 : xbsIndex_r4/Slice  nbits=sample_width  boolean_output=off  mode=Upper Bit Location + Width  bit1=-5*sample_width  base1=MSB of Input  bit0=0  base0=LSB of Input  dbl_ovrd=off  block_type=slice
      settings: block_version=11.3
  Slice6 : xbsIndex_r4/Slice  nbits=sample_width  boolean_output=off  mode=Upper Bit Location + Width  bit1=-6*sample_width  base1=MSB of Input  bit0=0  base0=LSB of Input  dbl_ovrd=off  block_type=slice
      settings: block_version=11.3
  Slice7 : xbsIndex_r4/Slice  nbits=sample_width  boolean_output=off  mode=Upper Bit Location + Width  bit1=-7*sample_width  base1=MSB of Input  bit0=0  base0=LSB of Input  dbl_ovrd=off  block_type=slice
      settings: block_version=11.3
  wires:
  Gateway Out8/1 -> Scope/2
  Sync/1 -> Gateway Out8/1
  Multiport Switch/1 -> Scope/1
  Gateway Out7/1 -> Multiport Switch/9
  Gateway Out6/1 -> Multiport Switch/8
  Gateway Out5/1 -> Multiport Switch/7
  Gateway Out4/1 -> Multiport Switch/6
  Gateway Out3/1 -> Multiport Switch/5
  Gateway Out2/1 -> Multiport Switch/4
  Gateway Out1/1 -> Multiport Switch/3
  Gateway Out/1 -> Multiport Switch/2
  Counter Free-Running/1 -> Multiport Switch/1
  Slice7/1 -> Gateway Out7/1
  Slice6/1 -> Gateway Out6/1
  Slice5/1 -> Gateway Out5/1
  Slice4/1 -> Gateway Out4/1
  Slice3/1 -> Gateway Out3/1
  Slice2/1 -> Gateway Out2/1
  Slice1/1 -> Gateway Out1/1
  Slice/1 -> Gateway Out/1
  In1/1 -> Slice7/1, Slice6/1, Slice5/1, Slice4/1, Slice3/1, Slice2/1, Slice1/1, Slice/1
